simulink model "HeightDistributedThermalMass"  (R2024b)
settings: Solver=VariableStepAuto  StartTime=0.0  StopTime=1000  RelTol=1e-4
libraries: fl_lib x17, nesl_utility x7, batt_lib x2
settings Model: Creator=xiangchz  LastModifiedBy=xiangchz

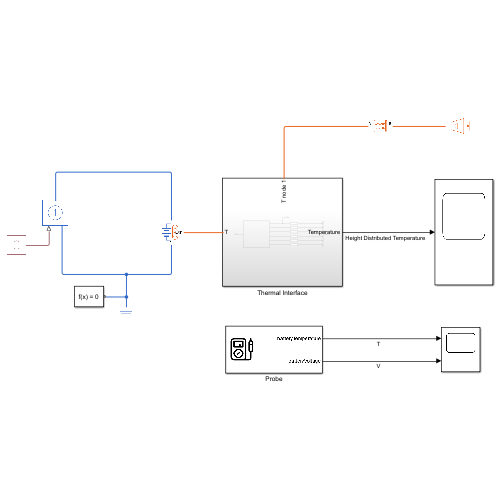
[thumbnail: Simulink's stored preview of the top-level diagram]
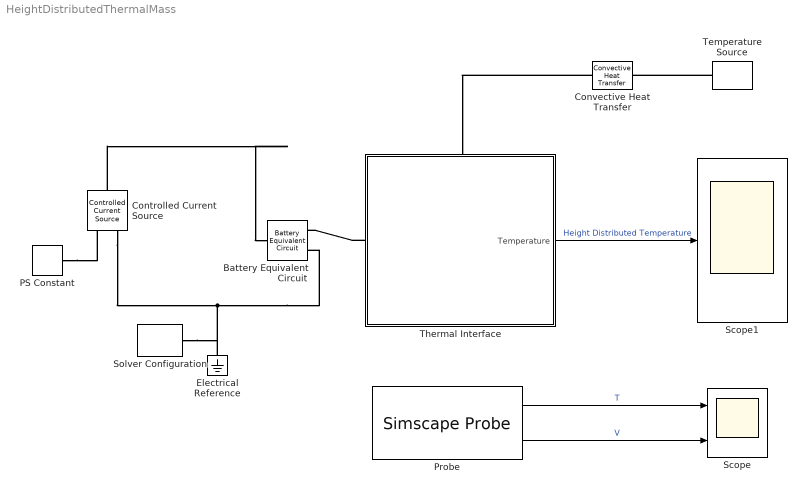
== system HeightDistributedThermalMass ==
  Battery Equivalent Circuit : batt_lib/Cells/Battery Equivalent Circuit  BatteryCapacity=27 A*hr  ThermalModel=simscape.battery.enum.cells.BatteryThermalModel.HeightDistributedMass  ExtrapolationMethod=simscape.enum.extrapolation.nearest  SOCBreakpoints=[0, .1, .25, .5, .75, .9, 1]  TemperatureBreakpoints=[278, 293, 313] K  OpenCircuitVoltage=[3.5057, 3.566, 3.6337, 3.7127, 3.9259, 4.0777, 4.1928] V  OpenCircuitVoltageThermal=[3.49, 3.5, 3.51; 3.55, 3.57, 3.56; 3.62, 3.63, 3.64; 3.71, 3.71, 3.72; 3.91, 3.93, 3.94; 4.07, 4.08, 4.08; 4.19, 4.19, 4.19] V  VoltageRange=[0, inf] V  HysteresisModel=simscape.battery.enum.cells.HysteresisModel.none  MaximumHysteresisVoltage=[0, 0, 0, 0, 0, 0, 0] V  InstantaneousHysteresisVoltage=[0, 0, 0, 0, 0, 0, 0] V  HysteresisRate=0.1  MaximumHysteresisVoltageThermal=[0, 0, 0; 0, 0, 0; 0, 0, 0; 0, 0, 0; 0, 0, 0; 0, 0, 0; 0, 0, 0] V  InstantaneousHysteresisVoltageThermal=[0, 0, 0; 0, 0, 0; 0, 0, 0; 0, 0, 0; 0, 0, 0; 0, 0, 0; 0, 0, 0] V  HysteresisRateThermal=0.1  ResistanceSOCBreakpoints=[0, .1, .25, .5, .75, .9, 1]  ResistanceTemperatureBreakpoints=[278, 293, 313] K  CurrentDirectionality=simscape.battery.enum.cells.BatteryEnable.Disabled  R0=[.0085, .0085, .0087, .0082, .0083, .0085, .0085] Ohm  R0Thermal=[.0117, .0085, .009; .011, .0085, .009; .0114, .0087, .0092; .0107, .0082, .0088; .0107, .0083, .0091; .0113, .0085, .0089; .0116, .0085, .0089] Ohm  DischargeR0=[.0085, .0085, .0087, .0082, .0083, .0085, .0085] Ohm  ChargeR0=[.0085, .0085, .0087, .0082, .0083, .0085, .0085] Ohm  ChargeR0Thermal=[.0117, .0085, .009; .011, .0085, .009; .0114, .0087, .0092; .0107, .0082, .0088; .0107, .0083, .0091; .0113, .0085, .0089; .0116, .0085, .0089] Ohm  DischargeR0Thermal=[.0117, .0085, .009; .011, .0085, .009; .0114, .0087, .0092; .0107, .0082, .0088; .0107, .0083, .0091; .0113, .0085, .0089; .0116, .0085, .0089] Ohm  SelfDischargeResistor=simscape.battery.enum.cells.BatteryEnable.Disabled  SelfDischargeR=7e3 Ohm  SelfDischargeRThermal=[8000, 7000, 6000] Ohm  RCPairs=simscape.battery.enum.cells.RCPairs.noDynamics  R1=[.0029, .0024, .0026, .0016, .0023, .0018, .0017] Ohm  Tau1=[36, 45, 105, 29, 77, 33, 39] s  R2=[.0029, .0024, .0026, .0016, .0023, .0018, .0017] Ohm  Tau2=[36, 45, 105, 29, 77, 33, 39] s  R3=[.0029, .0024, .0026, .0016, .0023, .0018, .0017] Ohm  Tau3=[36, 45, 105, 29, 77, 33, 39] s  DischargeR1=[.0029, .0024, .0026, .0016, .0023, .0018, .0017] Ohm  DischargeTau1=[36, 45, 105, 29, 77, 33, 39] s  ChargeR1=[.0029, .0024, .0026, .0016, .0023, .0018, .0017] Ohm  ChargeTau1=[36, 45, 105, 29, 77, 33, 39] s  DischargeR2=[.0029, .0024, .0026, .0016, .0023, .0018, .0017] Ohm  DischargeTau2=[36, 45, 105, 29, 77, 33, 39] s  ChargeR2=[.0029, .0024, .0026, .0016, .0023, .0018, .0017] Ohm  ChargeTau2=[36, 45, 105, 29, 77, 33, 39] s  DischargeR3=[.0029, .0024, .0026, .0016, .0023, .0018, .0017] Ohm  DischargeTau3=[36, 45, 105, 29, 77, 33, 39] s  ChargeR3=[.0029, .0024, .0026, .0016, .0023, .0018, .0017] Ohm  ChargeTau3=[36, 45, 105, 29, 77, 33, 39] s  R1Thermal=[.0109, .0029, .0013; .0069, .0024, .0012; .0047, .0026, .0013; .0034, .0016, .001; .0033, .0023, .0014; .0033, .0018, .0011; .0028, .0017, .0011] Ohm  Tau1Thermal=[20, 36, 39; 31, 45, 39; 109, 105, 61; 36, 29, 26; 59, 77, 67; 40, 33, 29; 25, 39, 33] s  R2Thermal=[.0109, .0029, .0013; .0069, .0024, .0012; .0047, .0026, .0013; .0034, .0016, .001; .0033, .0023, .0014; .0033, .0018, .0011; .0028, .0017, .0011] Ohm  Tau2Thermal=[20, 36, 39; 31, 45, 39; 109, 105, 61; 36, 29, 26; 59, 77, 67; 40, 33, 29; 25, 39, 33] s  R3Thermal=[.0109, .0029, .0013; .0069, .0024, .0012; .0047, .0026, .0013; .0034, .0016, .001; .0033, .0023, .0014; .0033, .0018, .0011; .0028, .0017, .0011] Ohm  Tau3Thermal=[20, 36, 39; 31, 45, 39; 109, 105, 61; 36, 29, 26; 59, 77, 67; 40, 33, 29; 25, 39, 33] s  DischargeR1Thermal=[.0109, .0029, .0013; .0069, .0024, .0012; .0047, .0026, .0013; .0034, .0016, .001; .0033, .0023, .0014; .0033, .0018, .0011; .0028, .0017, .0011] Ohm  DischargeTau1Thermal=[20, 36, 39; 31, 45, 39; 109, 105, 61; 36, 29, 26; 59, 77, 67; 40, 33, 29; 25, 39, 33] s  ChargeR1Thermal=[.0109, .0029, .0013; .0069, .0024, .0012; .0047, .0026, .0013; .0034, .0016, .001; .0033, .0023, .0014; .0033, .0018, .0011; .0028, .0017, .0011] Ohm  ChargeTau1Thermal=[20, 36, 39; 31, 45, 39; 109, 105, 61; 36, 29, 26; 59, 77, 67; 40, 33, 29; 25, 39, 33] s  DischargeR2Thermal=[.0109, .0029, .0013; .0069, .0024, .0012; .0047, .0026, .0013; .0034, .0016, .001; .0033, .0023, .0014; .0033, .0018, .0011; .0028, .0017, .0011] Ohm  DischargeTau2Thermal=[20, 36, 39; 31, 45, 39; 109, 105, 61; 36, 29, 26; 59, 77, 67; 40, 33, 29; 25, 39, 33] s  ChargeR2Thermal=[.0109, .0029, .0013; .0069, .0024, .0012; .0047, .0026, .0013; .0034, .0016, .001; .0033, .0023, .0014; .0033, .0018, .0011; .0028, .0017, .0011] Ohm  ChargeTau2Thermal=[20, 36, 39; 31, 45, 39; 109, 105, 61; 36, 29, 26; 59, 77, 67; 40, 33, 29; 25, 39, 33] s  DischargeR3Thermal=[.0109, .0029, .0013; .0069, .0024, .0012; .0047, .0026, .0013; .0034, .0016, .001; .0033, .0023, .0014; .0033, .0018, .0011; .0028, .0017, .0011] Ohm  DischargeTau3Thermal=[20, 36, 39; 31, 45, 39; 109, 105, 61; 36, 29, 26; 59, 77, 67; 40, 33, 29; 25, 39, 33] s  ChargeR3Thermal=[.0109, .0029, .0013; .0069, .0024, .0012; .0047, .0026, .0013; .0034, .0016, .001; .0033, .0023, .0014; .0033, .0018, .0011; .0028, .0017, .0011] Ohm  ChargeTau3Thermal=[20, 36, 39; 31, 45, 39; 109, 105, 61; 36, 29, 26; 59, 77, 67; 40, 33, 29; 25, 39, 33] s  CyclingAgingMethod=simscape.battery.enum.cells.CyclingAgingMethod.disabled  NumDisCycles=100  OCVChange=0  R0Change=0  CapacityChange=0  SelfDischargeRChange=0  R1Change=0  R2Change=0  R3Change=0  NumDisCyclesBreakpoints=[0, 100, 200, 300]  AgingTemperatureBreakpoints=[298.15, 323.15] K  OCVChangeVec=[0, 0, 0, 0]  R0ChangeVec=[0, 0, 0, 0]  CapacityChangeVec=[0, 0, 0, 0]  SelfDischargeRChangeVec=[0, 0, 0, 0]  R1ChangeVec=[0, 0, 0, 0]  R2ChangeVec=[0, 0, 0, 0]  R3ChangeVec=[0, 0, 0, 0]  OCVChangeThermal=[0, 0; 0, 0; 0, 0; 0, 0]  R0ChangeThermal=[0, 0; 0, 0; 0, 0; 0, 0]  CapacityChangeThermal=[0, 0; 0, 0; 0, 0; 0, 0]  SelfDischargeRChangeThermal=[0, 0; 0, 0; 0, 0; 0, 0]  R1ChangeThermal=[0, 0; 0, 0; 0, 0; 0, 0]  R2ChangeThermal=[0, 0; 0, 0; 0, 0; 0, 0]  R3ChangeThermal=[0, 0; 0, 0; 0, 0; 0, 0]  CalendarAgeResistance=simscape.battery.enum.cells.BatteryEnable.Disabled  CalendarAgeCapacity=simscape.battery.enum.cells.BatteryEnable.Disabled  CalendarAgingMethod=simscape.battery.enum.cells.CalendarAgingMethod.equation  StorageVariable=simscape.battery.enum.cells.StorageVariable.OCV  OCVDuringStorage=0.9  SOCDuringStorage=0.6  StorageTimeIntervals=[0] d  StorageTemperatures=[273] K  ResistanceScalingOCV=2.2134e6  ResistanceScalingOCVOffset=1.632e6  ResistanceExponentialIncrease=0.515833569 V  ResistanceTimeExponent=0.75  ResistanceAgeTemperatureBreakpoints=[273.15, 298.15, 323.15] K  ResistanceAgeTimeBreakpoints=[0, 90, 180, 270] d  PercentResistanceChange=[0, 0, 0]  ResistanceTimeBreakpoints=100 d  PercentResistanceChangeThermal=[0, 0, 0; 0, 0, 0; 0, 0, 0; 0, 0, 0]  CapacityScalingOCV=1.5097e07  CapacityScalingOCVOffset=8.3625e06  CapacityExponentialIncrease=0.6011 V  CapacityTimeExponent=0.75  CapacityAgeTemperatureBreakpoints=[273.15, 298.15, 323.15] K  CapacityAgeTimeBreakpoints=[0, 90, 180, 270] d  PercentCapacityChange=[0, 0, 0]  CapacityTimeBreakpoints=100 d  PercentCapacityChangeThermal=[0, 0, 0; 0, 0, 0; 0, 0, 0; 0, 0, 0]  SimulationTemperature=298.15 K  BatteryThermalMass=100 J/K  NumThermalModels=6  ThermalConductivityZ=18 W/(K*m)  CrossSectionalAreaXY=3.5e-4 m^2  Height=0.07 m  ReversibleHeatModel=simscape.battery.enum.cells.ReversibleHeatModel.Disabled  EntropicCoefficient=[0, 0, 0, 0, 0, 0, 0] mV/K  stateOfCharge_specify=off  stateOfCharge_priority=High  stateOfCharge=1  stateOfCharge_nominal_specify=off  stateOfCharge_nominal_value=1  stateOfCharge_nominal_unit=1  numCycles_specify=off  numCycles_priority=High  numCycles=0  numCycles_nominal_specify=off  numCycles_nominal_value=1  numCycles_nominal_unit=1  batteryVoltage_specify=off  batteryVoltage_priority=None  batteryVoltage=0 V  batteryVoltage_nominal_specify=off  batteryVoltage_nominal_value=1  batteryVoltage_nominal_unit=V  batteryCurrent_specify=off  batteryCurrent_priority=None  batteryCurrent=0 A  batteryCurrent_nominal_specify=off  batteryCurrent_nominal_value=1  batteryCurrent_nominal_unit=A  batteryTemperature_specify=off  batteryTemperature_priority=High  batteryTemperature=298.15 K  batteryTemperature_nominal_specify=off  batteryTemperature_nominal_value=1  batteryTemperature_nominal_unit=K  hysteresisState_specify=off  hysteresisState_priority=High  hysteresisState=0  hysteresisState_nominal_specify=off  hysteresisState_nominal_value=1  hysteresisState_nominal_unit=1  isExothermFaulted_specify=off  isExothermFaulted_priority=None  isExothermFaulted=0  isExothermFaulted_nominal_specify=off  isExothermFaulted_nominal_value=1  isExothermFaulted_nominal_unit=1  reactionHeatRate_specify=off  reactionHeatRate_priority=None  reactionHeatRate=0 W  reactionHeatRate_nominal_specify=off  reactionHeatRate_nominal_value=1  reactionHeatRate_nominal_unit=W  reactionExtent_specify=off  reactionExtent_priority=None  reactionExtent=0  reactionExtent_nominal_specify=off  reactionExtent_nominal_value=1  reactionExtent_nominal_unit=1
      settings: InternalSimscapePortConfiguration="{\"Bottom\":[{\"id\":\"n\",\"label\":\"-\",\"type\":\"foundation.electrical.electrical\"}],\"Left\":[],\"Right\":[{\"id\":\"HDistributed\",\"label\":\"HDist\",\"type\":\"foundation.thermal.thermal\"}],\"Top\":[{\"id\":\"p\",\"label\":\"+\",\"type\":\"foundation.electrical.electrical\"}]}"
  Controlled Current Source : fl_lib/Electrical/Electrical Sources/Controlled Current Source
  Convective Heat Transfer : fl_lib/Thermal/Thermal Elements/Convective Heat Transfer  thermal_type=foundation.enum.constant_variable.constant  area=50 cm^2  heat_tr_coeff=100 W/(K*m^2)  min_heat_tr_coeff=1e-3 W/(K*m^2)  T_specify=off  T_priority=None  T=0 K  T_nominal_specify=off  T_nominal_value=1  T_nominal_unit=K  Q_specify=off  Q_priority=None  Q=0 W  Q_nominal_specify=off  Q_nominal_value=1  Q_nominal_unit=W
  Electrical Reference : fl_lib/Electrical/Electrical Elements/Electrical Reference
  PS Constant : fl_lib/Physical Signals/Sources/PS Constant  constant=-27 A
  Probe : SimscapeProbe  BoundBlock=1  Variables="{\"batteryTemperature\":{\"Unit\":\"K\",\"PortLabel\":\"batteryTemperature\",\"Probing\":\"ON\"},\"batteryVoltage\":{\"Unit\":\"V\",\"PortLabel\":\"batteryVoltage\",\"Probing\":\"ON\"}}"
  Scope : Scope  NumInputPorts=2
  Scope1 : Scope
  Solver Configuration : nesl_utility/Solver Configuration  PhysicalDomain=network_engine_domain  SubClassName=solver  LeftPortType=input  RightPortType=generic  Tones=[]  Harmonics=[]  SimulateNoise=off  Profile=off  UseLocalSampling=off  EnableSwitchedLinearOptims=on  FrequencyDomain=off  UseCCode=off  RelTol=0.001  AbsTol=0.001  MinStep=1e-09  ToWorkspace=off  RevertToSquareIcSolve=off  NumHomotopyIterations=100  PhasorMode=off  PhasorModeNumHarmonics=1  ConsistencySolver=NEWTON_XTOL_AFTER_FTOL  IndexReductionMethod=DerivativeReplacement  DoDC=off  ResidualTolerance=1e-09  ConsistencyTolSource=GLOBAL  ConsistencyAbsTol=0.001  ConsistencyRelTol=0.001  ConsistencyTolFactor=0.001  UseLocalSolver=off  LocalSolverChoice=NE_BACKWARD_EULER_ADVANCER  ResolveIndetEquations=on  FunctionEvalNumThread=1  LocalSolverSampleTime=0.001  DoFixedCost=off  MaxNonlinIter=3  MaxModeIter=2  ComputeImpulses=off  ImpulseIterations=2  LinearAlgebra=auto  LinearAlgebraNumThread=0  EquationFormulation=NE_TIME_EF  DelaysMemoryBudget=1024  AutomaticFiltering=on  FilteringTimeConstant=0.001  PartitionStorageMethod=AS_NEEDED  PartitionMemoryBudget=1024  PartitionMethod=ROBUST  MultibodyUseLocalSolver=off  MultibodyLocalSolverChoice=ODE1  MultibodyLocalSolverSampleTime=0.001
  Temperature Source : fl_lib/Thermal/Thermal Sources/Temperature Source  temperature=293.15 K
  Thermal Interface : Subsystem
      settings: PortSchema="{\"entries\":[{\"content\":{\"sides\":[{\"content\":{\"connectorIds\":[\"LConn1\"]},\"type\":\"ConnectorPlacement.EquallySpacedRectSide\",\"uuid\":\"25488635-171d-4684-a7e4-a35c4d23970d\"},{\"content\":{\"connectorIds\":[\"Out1\"],\"side\":\"RIGHT\"},\"type\":\"ConnectorPlacement.EquallySpacedRectSide\",\"uuid\":\"438962aa-9c72-460f-b730-8b0e0500cc9a\"},{\"content\":{\"connectorIds\":[\"LConn2\"],\"side\":\"TOP\"},\"type\":\"ConnectorPlacement.EquallySpacedRectSide\",\"uuid\":\"c5322876-b4de-49ce-a17c-611fffbca7b6\"}]},\"type\":\"ConnectorPlacement.EquallySpacedConnector\",\"uuid\":\"b26e0eb7-8301-47a6-b5c4-a233b12059e4\"}],\"packageUris\":[\"http://schema.mathworks.com/mf0/Connector/R2020b\"],\"version\":\"1.0\"}"
  wires:
  Probe/1 -> Scope/1  "T"
  Probe/2 -> Scope/2  "V"
  Thermal Interface/1(Temperature) -> Scope1/1  "Height Distributed Temperature"
  connections:
  Controlled Current Source/LConn1 -- Battery Equivalent Circuit/LConn1
  Controlled Current Source/RConn2 -- Battery Equivalent Circuit/RConn2 -- Solver Configuration/RConn1 -- Electrical Reference/LConn1
  PS Constant/RConn1 -- Controlled Current Source/RConn1
  Temperature Source/LConn1 -- Convective Heat Transfer/RConn1
  Convective Heat Transfer/LConn1 -- Thermal Interface/LConn2
  Thermal Interface/LConn1 -- Battery Equivalent Circuit/RConn1

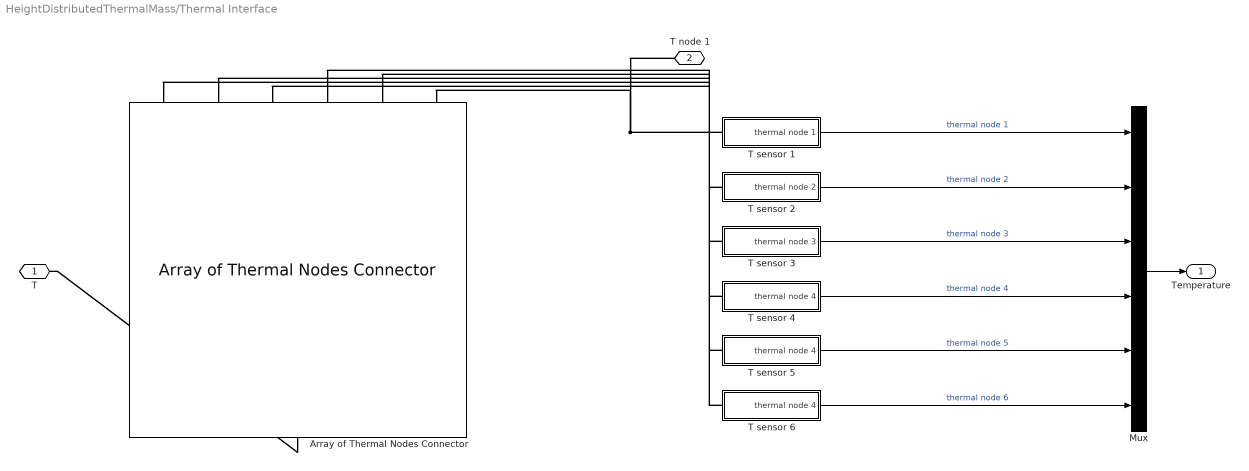
== system HeightDistributedThermalMass/Thermal Interface ==
  Array of Thermal Nodes Connector : batt_lib/Thermal/Array of Thermal Nodes Connector  numInputConnections=simscape.battery.enum.thermal.numArrayOfNodesConnections.six  concatenateDimension=1  complementaryDimensionsSize=1  inNode1NumElements=1  inNode2NumElements=1  inNode3NumElements=1  inNode4NumElements=1  inNode5NumElements=1  inNode6NumElements=1  inNode7NumElements=1  inNode8NumElements=1  inNode9NumElements=1  inNode10NumElements=1  inNode11NumElements=1  inNode12NumElements=1  inNode13NumElements=1  inNode14NumElements=1  inNode15NumElements=1  inNode16NumElements=1  inNode17NumElements=1  inNode18NumElements=1  inNode19NumElements=1  inNode20NumElements=1  inNode21NumElements=1  inNode22NumElements=1  inNode23NumElements=1  inNode24NumElements=1  inNode25NumElements=1  inNode26NumElements=1  inNode27NumElements=1  inNode28NumElements=1  inNode29NumElements=1  inNode30NumElements=1  inNode31NumElements=1  inNode32NumElements=1  inNode33NumElements=1  inNode34NumElements=1  inNode35NumElements=1  inNode36NumElements=1  inNode37NumElements=1  inNode38NumElements=1  inNode39NumElements=1  inNode40NumElements=1  inNode41NumElements=1  inNode42NumElements=1  inNode43NumElements=1  inNode44NumElements=1  inNode45NumElements=1  inNode46NumElements=1  inNode47NumElements=1  inNode48NumElements=1  inNode49NumElements=1  inNode50NumElements=1
      settings: InternalSimscapePortConfiguration="{\"Bottom\":[{\"id\":\"outConn\",\"label\":\"outConn\",\"type\":\"foundation.thermal.thermal\"}],\"Left\":[],\"Right\":[],\"Top\":[{\"id\":\"inConn1\",\"label\":\"inConn1\",\"type\":\"foundation.thermal.thermal\"},{\"id\":\"inConn2\",\"label\":\"inConn2\",\"type\":\"foundation.thermal.thermal\"},{\"id\":\"inConn3\",\"label\":\"inConn3\",\"type\":\"foundation.thermal.thermal\"},{\"id\":\"inConn4\",\"label\":\"inConn4\",\"type\":\"foundation.thermal.thermal\"},{\"id\":\"inConn5\",\"label\":\"inConn5\",\"type\":\"foundation.thermal.thermal\"},{\"id\":\"inConn6\",\"label\":\"inConn6\",\"type\":\"foundation.thermal.thermal\"}]}"
  Mux : Mux  Inputs=6
  T sensor 1 : Subsystem
  T sensor 2 : Subsystem
  T sensor 3 : Subsystem
  T sensor 4 : Subsystem
  T sensor 5 : Subsystem
  T sensor 6 : Subsystem
  T : PMIOPort  Side=Left
  T node 1 : PMIOPort  Port=2  Side=Left
  Temperature : Outport
  wires:
  T sensor 2/1(thermal node 2) -> Mux/2  "thermal node 2"
  T sensor 3/1(thermal node 3) -> Mux/3  "thermal node 3"
  T sensor 1/1(thermal node 1) -> Mux/1  "thermal node 1"
  T sensor 4/1(thermal node 4) -> Mux/4  "thermal node 4"
  T sensor 6/1(thermal node 4) -> Mux/6  "thermal node 6"
  T sensor 5/1(thermal node 4) -> Mux/5  "thermal node 5"
  Mux/1 -> Temperature/1
  connections:
  T sensor 1/LConn1 -- T node 1/RConn1 -- Array of Thermal Nodes Connector/LConn1
  T sensor 4/LConn1 -- Array of Thermal Nodes Connector/LConn4
  T sensor 6/LConn1 -- Array of Thermal Nodes Connector/LConn6
  Array of Thermal Nodes Connector/RConn1 -- T/RConn1
  T sensor 5/LConn1 -- Array of Thermal Nodes Connector/LConn5
  T sensor 2/LConn1 -- Array of Thermal Nodes Connector/LConn2
  T sensor 3/LConn1 -- Array of Thermal Nodes Connector/LConn3

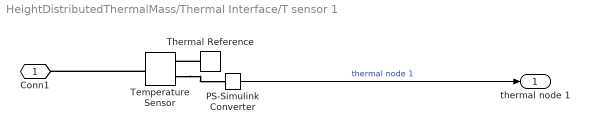
== system HeightDistributedThermalMass/Thermal Interface/T sensor 1 ==
  PS-Simulink Converter : nesl_utility/PS-Simulink Converter  PhysicalDomain=network_engine_domain  SubClassName=ps_output  LeftPortType=input  RightPortType=output  PseudoPeriodic=off  Frequencies=[]  VectorFormat=inherit  Unit=inherit  AffineConversion=off
  Temperature Sensor : fl_lib/Thermal/Thermal Sensors/Temperature Sensor  temperature_measure=foundation.enum.MeasurementReference.difference
  Thermal Reference : fl_lib/Thermal/Thermal Elements/Thermal Reference
  Conn1 : PMIOPort  Side=Left
  thermal node 1 : Outport
  wires:
  PS-Simulink Converter/1 -> thermal node 1/1  "thermal node 1"
  connections:
  Temperature Sensor/RConn2 -- PS-Simulink Converter/LConn1
  Thermal Reference/LConn1 -- Temperature Sensor/RConn1
  Temperature Sensor/LConn1 -- Conn1/RConn1

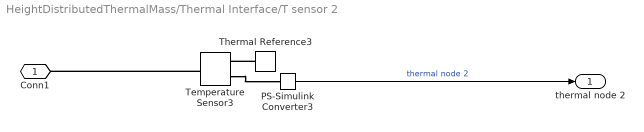
== system HeightDistributedThermalMass/Thermal Interface/T sensor 2 ==
  PS-Simulink Converter3 : nesl_utility/PS-Simulink Converter  PhysicalDomain=network_engine_domain  SubClassName=ps_output  LeftPortType=input  RightPortType=output  PseudoPeriodic=off  Frequencies=[]  VectorFormat=inherit  Unit=inherit  AffineConversion=off
  Temperature Sensor3 : fl_lib/Thermal/Thermal Sensors/Temperature Sensor  temperature_measure=foundation.enum.MeasurementReference.difference
  Thermal Reference3 : fl_lib/Thermal/Thermal Elements/Thermal Reference
  Conn1 : PMIOPort  Side=Left
  thermal node 2 : Outport
  wires:
  PS-Simulink Converter3/1 -> thermal node 2/1  "thermal node 2"
  connections:
  Temperature Sensor3/RConn2 -- PS-Simulink Converter3/LConn1
  Thermal Reference3/LConn1 -- Temperature Sensor3/RConn1
  Temperature Sensor3/LConn1 -- Conn1/RConn1

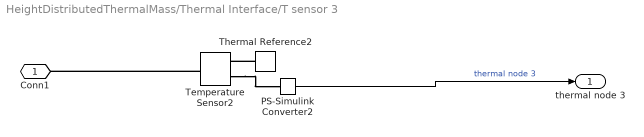
== system HeightDistributedThermalMass/Thermal Interface/T sensor 3 ==
  PS-Simulink Converter2 : nesl_utility/PS-Simulink Converter  PhysicalDomain=network_engine_domain  SubClassName=ps_output  LeftPortType=input  RightPortType=output  PseudoPeriodic=off  Frequencies=[]  VectorFormat=inherit  Unit=inherit  AffineConversion=off
  Temperature Sensor2 : fl_lib/Thermal/Thermal Sensors/Temperature Sensor  temperature_measure=foundation.enum.MeasurementReference.difference
  Thermal Reference2 : fl_lib/Thermal/Thermal Elements/Thermal Reference
  Conn1 : PMIOPort  Side=Left
  thermal node 3 : Outport
  wires:
  PS-Simulink Converter2/1 -> thermal node 3/1  "thermal node 3"
  connections:
  Temperature Sensor2/RConn2 -- PS-Simulink Converter2/LConn1
  Thermal Reference2/LConn1 -- Temperature Sensor2/RConn1
  Temperature Sensor2/LConn1 -- Conn1/RConn1

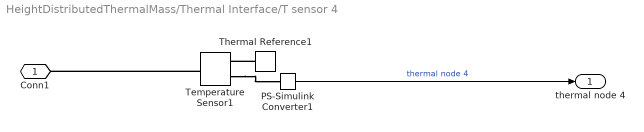
== system HeightDistributedThermalMass/Thermal Interface/T sensor 4 ==
  PS-Simulink Converter1 : nesl_utility/PS-Simulink Converter  PhysicalDomain=network_engine_domain  SubClassName=ps_output  LeftPortType=input  RightPortType=output  PseudoPeriodic=off  Frequencies=[]  VectorFormat=inherit  Unit=inherit  AffineConversion=off
  Temperature Sensor1 : fl_lib/Thermal/Thermal Sensors/Temperature Sensor  temperature_measure=foundation.enum.MeasurementReference.difference
  Thermal Reference1 : fl_lib/Thermal/Thermal Elements/Thermal Reference
  Conn1 : PMIOPort  Side=Left
  thermal node 4 : Outport
  wires:
  PS-Simulink Converter1/1 -> thermal node 4/1  "thermal node 4"
  connections:
  Thermal Reference1/LConn1 -- Temperature Sensor1/RConn1
  Temperature Sensor1/RConn2 -- PS-Simulink Converter1/LConn1
  Temperature Sensor1/LConn1 -- Conn1/RConn1

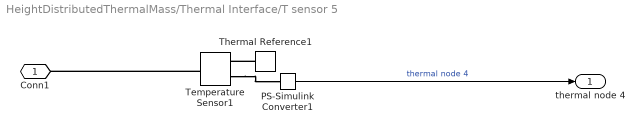
== system HeightDistributedThermalMass/Thermal Interface/T sensor 5 ==
  PS-Simulink Converter1 : nesl_utility/PS-Simulink Converter  PhysicalDomain=network_engine_domain  SubClassName=ps_output  LeftPortType=input  RightPortType=output  PseudoPeriodic=off  Frequencies=[]  VectorFormat=inherit  Unit=inherit  AffineConversion=off
  Temperature Sensor1 : fl_lib/Thermal/Thermal Sensors/Temperature Sensor  temperature_measure=foundation.enum.MeasurementReference.difference
  Thermal Reference1 : fl_lib/Thermal/Thermal Elements/Thermal Reference
  Conn1 : PMIOPort  Side=Left
  thermal node 4 : Outport
  wires:
  PS-Simulink Converter1/1 -> thermal node 4/1  "thermal node 4"
  connections:
  Temperature Sensor1/LConn1 -- Conn1/RConn1
  Temperature Sensor1/RConn2 -- PS-Simulink Converter1/LConn1
  Thermal Reference1/LConn1 -- Temperature Sensor1/RConn1

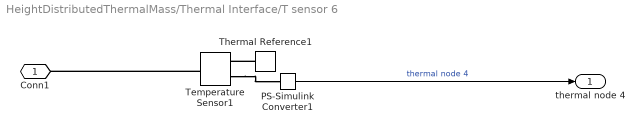
== system HeightDistributedThermalMass/Thermal Interface/T sensor 6 ==
  PS-Simulink Converter1 : nesl_utility/PS-Simulink Converter  PhysicalDomain=network_engine_domain  SubClassName=ps_output  LeftPortType=input  RightPortType=output  PseudoPeriodic=off  Frequencies=[]  VectorFormat=inherit  Unit=inherit  AffineConversion=off
  Temperature Sensor1 : fl_lib/Thermal/Thermal Sensors/Temperature Sensor  temperature_measure=foundation.enum.MeasurementReference.difference
  Thermal Reference1 : fl_lib/Thermal/Thermal Elements/Thermal Reference
  Conn1 : PMIOPort  Side=Left
  thermal node 4 : Outport
  wires:
  PS-Simulink Converter1/1 -> thermal node 4/1  "thermal node 4"
  connections:
  Thermal Reference1/LConn1 -- Temperature Sensor1/RConn1
  Temperature Sensor1/RConn2 -- PS-Simulink Converter1/LConn1
  Temperature Sensor1/LConn1 -- Conn1/RConn1
